simulink model "Sist_stab_n"  (R2018b)
settings: Solver=VariableStepAuto  StartTime=0.0  StopTime=10.0  RelTol=1e-3
settings Model: Creator=Танечка  LastModifiedBy=Танечка

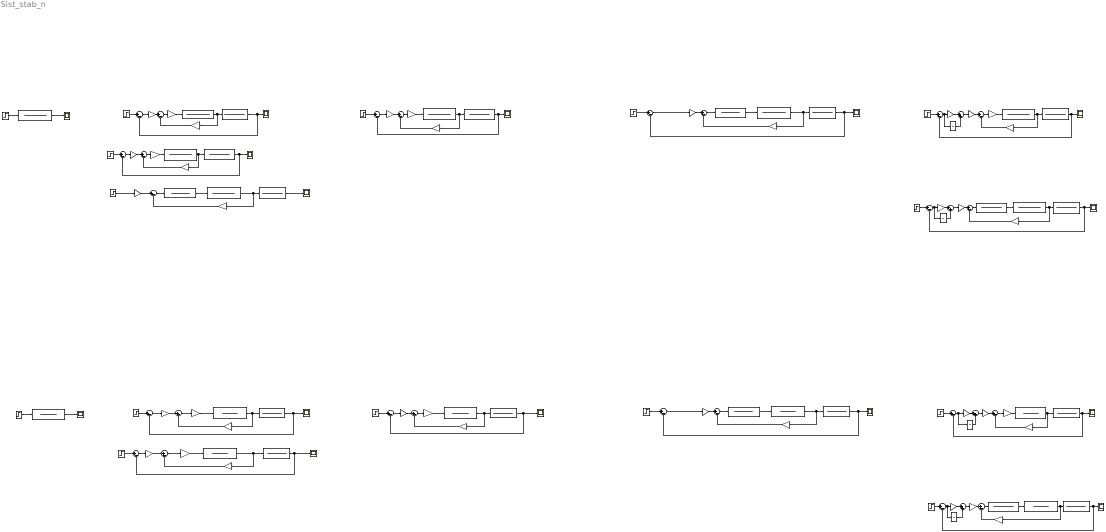
== system Sist_stab_n ==
  note: Скорость 1: V=650
  note: Обьект
  note: С ПИ-регулятором
  note: Подбор с двигателем
  note: Подбор позиционной ОС
  note: $n_{y\ тек}$
  note: $\omega_{ z}$
  note: $\delta$
  note: $\Delta$
  note: $Ф_{ рп}$
  note: $n_{y\ тек}$
  note: $K_{ \dot\theta}$
  note: $n_{y\ зад}$
  note: $K_{ \dot\theta}$
  note: $n_{y\ тек}$
  note: $n_{y\ тек}$
  note: $Ф_{ рп}$
  note: $\omega_{ z}$
  note: $\Delta$
  note: $\delta$
  note: $n_{y\ зад}$
  note: $\omega_{ z}$
  note: $Ф_{ рп}$
  note: $n_{y\ тек}$
  note: $K_{ \dot\theta}$
  note: $\delta$
  note: $n_{y\ зад}$
  note: $n_{y\ тек}$
  note: $\Delta$
  note: $Ф_{ рп}$
  note: $\delta$
  note: $n_{y\ зад}$
  note: $K_{ \dot\theta}$
  note: $\Delta$
  note: $n_{y\ тек}$
  note: $n_{y\ тек}$
  note: $\omega_{ z}$
  note: $Ф_{ рп}$
  note: $n_{y\ тек}$
  note: $n_{y\ тек}$
  note: $\delta$
  note: $n_{y\ зад}$
  note: $\omega_{ z}$
  note: $K_{ \dot\theta}$
  note: $\Delta$
  note: $K_{ \dot\theta}$
  note: $\omega_{ z}$
  note: $\Delta$
  note: $n_{y\ тек}$
  note: $n_{y\ зад}$
  note: $Ф_{ рп}$
  note: $n_{y\ тек}$
  note: $\delta$
  note: Подбор скоростной ОС
  note: $K_{ \dot\theta}$
  note: $Ф_{ рп}$
  note: $\omega_{ z}$
  note: $n_{y\ тек}$
  note: $\delta$
  note: $n_{y\ зад}$
  note: $\Delta$
  note: $n_{y\ тек}$
  note: С ПИ-регулятором и двигателем
  note: $\delta$
  note: $n_{y\ тек}$
  note: $\Delta$
  note: $n_{y\ зад}$
  note: $n_{y\ тек}$
  note: $n_{y\ тек}$
  note: $n_{y\ тек}$
  note: $Ф_{ рп}$
  note: $\omega_{ z}$
  note: $n_{y\ зад}$
  note: $\omega_{ z}$
  note: $K_{ \dot\theta}$
  note: $n_{y\ зад}$
  note: $\omega_{ z}$
  note: $\omega_{ z}$
  note: $\delta$
  note: $\omega_{ z}$
  note: $n_{y\ тек}$
  note: $K_{ \dot\theta}$
  note: $\Delta$
  note: $n_{y\ тек}$
  note: $Ф_{ рп}$
  note: $\delta$
  note: $n_{y\ тек}$
  note: $\delta$
  note: $n_{y\ зад}$
  note: $\Delta$
  note: $Ф_{ рп}$
  note: $\Delta$
  note: $Ф_{ рп}$
  note: $n_{y\ зад}$
  note: $K_{ \dot\theta}$
  note: $K_{ \dot\theta}$
  note: С ПИ-регулятором и двигателем
  note: Подбор с двигателем
  note: С ПИ-регулятором
  note: $n_{y\ тек}$
  note: $\Delta$
  note: Обьект
  note: $\delta$
  note: $n_{y\ тек}$
  note: $n_{y\ тек}$
  note: $K_{ \dot\theta}$
  note: $\omega_{ z}$
  note: $Ф_{ рп}$
  note: $n_{y\ зад}$
  note: $\Delta$
  note: Подбор позиционной ОС
  note: $\delta$
  note: $Ф_{ рп}$
  note: $n_{y\ тек}$
  note: Подбор скоростной ОС
  note: $n_{y\ тек}$
  note: $K_{ \dot\theta}$
  note: Скорость 2: V=307
  note: $\mu$
  note: $\mu$
  Gain : Gain  Gain=5
  Gain{1,13,21,25} (4 alike) : Gain  Gain=10
  Gain10 : Gain  Gain=5
  Gain11 : Gain  Gain=0.4
  Gain{7,9,12,19,24,31,37,39} (8 alike) : Gain
  Gain{14,26,29,35} (4 alike) : Gain  Gain=0.25
  Gain15 : Gain  Gain=14
  Gain16 : Gain  Gain=0.2
  Gain17 : Gain  Gain=0.2
  Gain{8,18,30,38} (4 alike) : Gain  Gain=0.7
  Gain2 : Gain  Gain=14
  Gain22 : Gain  Gain=5
  Gain23 : Gain  Gain=0.4
  Gain27 : Gain  Gain=6
  Gain3 : Gain  Gain=0.01
  Gain32 : Gain  Gain=6
  Gain33 : Gain  Gain=0.01
  Gain{4,6,34,36} (4 alike) : Gain  Gain=0
  Gain5 : Gain  Gain=0.2
  Scope{,1..7,9..15} (15 alike) : Scope
  Step{,1..2,9..10} (5 alike) : Step  After=5  SampleTime=0
  Step{3..7,11..15} (10 alike) : Step  SampleTime=0
  Sum{1..9,12..16,19..23,25..30} (25 alike) : Sum  Inputs=|+-
  Sum{10..11,17..18} (4 alike) : Sum  Inputs=|++
  Transfer Fcn{,2,4,6,8,15,18} (7 alike) : TransferFcn  Numerator=[650]  Denominator="[57.3*9.81*1.75  57.3*9.81]"
  Transfer Fcn{1,3,5,7,10,14,16,19} (8 alike) : TransferFcn  Numerator=[0.42*1.75 0.42]  Denominator=[0.067*0.067 2*0.043*0.067 1]
  Transfer Fcn11 : TransferFcn  Numerator=[ 1]  Denominator=[0.005*0.005 2*0.7*0.005 1]
  Transfer Fcn{12,17,24,29} (4 alike) : TransferFcn  Denominator=[1 0]
  Transfer Fcn13 : TransferFcn  Numerator=[ 1]  Denominator=[0.01*0.01 2*0.7*0.01 1]
  Transfer Fcn{20..22,26..27,33,35} (7 alike) : TransferFcn  Numerator=[3*0.3 3]  Denominator=[0.1*0.1 2*0.2*0.1 1]
  Transfer Fcn23 : TransferFcn  Numerator=[ 1]  Denominator=[0.005*0.005 2*0.7*0.005 1]
  Transfer Fcn25 : TransferFcn  Numerator=[ 1]  Denominator=[0.01*0.01 2*0.7*0.01 1]
  Transfer Fcn{28,31..32,34,37..38} (6 alike) : TransferFcn  Numerator=[307]  Denominator="[57.3*9.81*0.3  57.3*9.81]"
  Transfer Fcn9 : TransferFcn  Numerator=[ 1]  Denominator=[0.01*0.01 2*0.7*0.01 1]
  wires:
  Sum3/1 -> Transfer Fcn9/1
  Gain/1 -> Sum3/1
  Transfer Fcn1/1 -> Gain16/1, Transfer Fcn/1
  Transfer Fcn/1 -> Scope/1
  Gain16/1 -> Sum3/2
  Step/1 -> Gain/1
  Transfer Fcn9/1 -> Transfer Fcn1/1
  Gain4/1 -> Sum2/2
  Step1/1 -> Sum1/1
  Transfer Fcn2/1 -> Scope1/1, Sum1/2
  Gain7/1 -> Transfer Fcn3/1
  Sum2/1 -> Gain7/1
  Transfer Fcn3/1 -> Transfer Fcn2/1, Gain4/1
  Gain1/1 -> Sum2/1
  Sum1/1 -> Gain1/1
  Sum5/1 -> Gain9/1
  Gain3/1 -> Sum5/1
  Transfer Fcn4/1 -> Scope2/1, Sum4/2
  Sum4/1 -> Gain3/1
  Gain9/1 -> Transfer Fcn5/1
  Gain6/1 -> Sum5/2
  Transfer Fcn5/1 -> Gain6/1, Transfer Fcn4/1
  Step2/1 -> Sum4/1
  Gain12/1 -> Transfer Fcn10/1
  Sum9/1 -> Gain12/1
  Step4/1 -> Sum8/1
  Gain10/1 -> Sum9/1
  Transfer Fcn8/1 -> Scope4/1, Sum8/2
  Sum8/1 -> Gain10/1
  Transfer Fcn10/1 -> Gain11/1, Transfer Fcn8/1
  Gain11/1 -> Sum9/2
  Transfer Fcn11/1 -> Transfer Fcn7/1
  Sum6/1 -> Transfer Fcn11/1
  Transfer Fcn7/1 -> Transfer Fcn6/1, Gain5/1
  Gain2/1 -> Sum6/1
  Gain5/1 -> Sum6/2
  Transfer Fcn6/1 -> Scope3/1, Sum7/2
  Step3/1 -> Sum7/1
  Sum10/1 -> Gain2/1
  Sum7/1 -> Transfer Fcn12/1, Gain8/1
  Transfer Fcn12/1 -> Sum10/2
  Gain8/1 -> Sum10/1
  Sum13/1 -> Gain13/1
  Gain14/1 -> Sum12/2
  Step5/1 -> Sum13/1
  Transfer Fcn16/1 -> Gain14/1, Transfer Fcn15/1
  Transfer Fcn13/1 -> Transfer Fcn16/1
  Sum12/1 -> Transfer Fcn13/1
  Gain13/1 -> Sum12/1
  Transfer Fcn15/1 -> Scope5/1, Sum13/2
  Sum15/1 -> Transfer Fcn17/1, Gain18/1
  Gain15/1 -> Sum14/1
  Sum14/1 -> Gain19/1
  Gain19/1 -> Transfer Fcn19/1
  Gain18/1 -> Sum11/1
  Transfer Fcn17/1 -> Sum11/2
  Transfer Fcn19/1 -> Transfer Fcn18/1, Gain17/1
  Transfer Fcn18/1 -> Scope6/1, Sum15/2
  Gain17/1 -> Sum14/2
  Sum11/1 -> Gain15/1
  Step6/1 -> Sum15/1
  Step7/1 -> Transfer Fcn14/1
  Transfer Fcn14/1 -> Scope7/1
  Transfer Fcn38/1 -> Scope11/1, Sum28/2
  Transfer Fcn20/1 -> Transfer Fcn32/1, Gain34/1
  Gain32/1 -> Sum27/1
  Transfer Fcn25/1 -> Transfer Fcn27/1
  Sum16/1 -> Gain21/1
  Sum19/1 -> Transfer Fcn25/1
  Transfer Fcn23/1 -> Transfer Fcn22/1
  Transfer Fcn24/1 -> Sum17/2
  Step10/1 -> Sum25/1
  Gain37/1 -> Transfer Fcn20/1
  Sum20/1 -> Gain25/1
  Sum29/1 -> Gain22/1
  Step9/1 -> Sum16/1
  Step12/1 -> Sum29/1
  Transfer Fcn34/1 -> Scope12/1, Sum29/2
  Step13/1 -> Sum20/1
  Transfer Fcn21/1 -> Transfer Fcn31/1, Gain36/1
  Gain24/1 -> Transfer Fcn33/1
  Transfer Fcn31/1 -> Sum25/2, Scope10/1
  Transfer Fcn33/1 -> Transfer Fcn34/1, Gain23/1
  Gain22/1 -> Sum30/1
  Transfer Fcn22/1 -> Transfer Fcn38/1, Gain35/1
  Sum17/1 -> Gain32/1
  Gain35/1 -> Sum27/2
  Step11/1 -> Sum28/1
  Sum26/1 -> Gain39/1
  Transfer Fcn27/1 -> Transfer Fcn37/1, Gain26/1
  Gain34/1 -> Sum23/2
  Gain36/1 -> Sum26/2
  Sum23/1 -> Gain37/1
  Sum30/1 -> Gain24/1
  Sum28/1 -> Transfer Fcn24/1, Gain38/1
  Transfer Fcn37/1 -> Scope13/1, Sum20/2
  Gain38/1 -> Sum17/1
  Gain25/1 -> Sum19/1
  Transfer Fcn26/1 -> Scope15/1
  Sum27/1 -> Transfer Fcn23/1
  Gain33/1 -> Sum26/1
  Step15/1 -> Transfer Fcn26/1
  Transfer Fcn32/1 -> Scope9/1, Sum16/2
  Gain26/1 -> Sum19/2
  Gain29/1 -> Sum21/2
  Sum18/1 -> Gain27/1
  Transfer Fcn35/1 -> Transfer Fcn28/1, Gain29/1
  Transfer Fcn29/1 -> Sum18/2
  Gain23/1 -> Sum30/2
  Transfer Fcn28/1 -> Scope14/1, Sum22/2
  Gain39/1 -> Transfer Fcn21/1
  Gain30/1 -> Sum18/1
  Sum22/1 -> Transfer Fcn29/1, Gain30/1
  Step14/1 -> Sum22/1
  Gain21/1 -> Sum23/1
  Gain31/1 -> Transfer Fcn35/1
  Sum25/1 -> Gain33/1
  Sum21/1 -> Gain31/1
  Gain27/1 -> Sum21/1
